simulink model "UZ_EnDat_be4_optimizing_agaib"  (R2023b)
settings: Solver=FixedStepDiscrete  StartTime=0  StopTime=0.002  RelTol=1e-3
model workspace (MAT data in the model file):
  Select = 0
libraries: hdlsllib x750, simulink x19, simulink_extras x4
(part 5 of 9)

== system UZ_EnDat_be4_optimizing_agaib/UZ_ENDAT/ManualSerialize/nibblepadding6/padding2 ==
  in : Inport
  Bit Shift2 : hdlsllib/Logic and Bit Operations/Bit Shift  mode=Shift Right Logical  N=1
  Bit Slice2 : hdlsllib/Logic and Bit Operations/Bit Slice  lidx=0  ridx=0
  Data Type Conversion2 : DataTypeConversion  OutDataTypeStr=boolean  RndMeth=Nearest  SaturateOnIntegerOverflow=off
  Switch2 : Switch  Criteria=u2 > Threshold  SaturateOnIntegerOverflow=off  InputSameDT=off
  out : Outport
  wires:
  in/1 -> Bit Shift2/1, Switch2/1, Bit Slice2/1
  Bit Shift2/1 -> Switch2/3
  Data Type Conversion2/1 -> Switch2/2
  Bit Slice2/1 -> Data Type Conversion2/1
  Switch2/1 -> out/1

== system UZ_EnDat_be4_optimizing_agaib/UZ_ENDAT/ManualSerialize/nibblepadding6/padding3 ==
  in : Inport
  Bit Shift2 : hdlsllib/Logic and Bit Operations/Bit Shift  mode=Shift Right Logical  N=1
  Bit Slice2 : hdlsllib/Logic and Bit Operations/Bit Slice  lidx=0  ridx=0
  Data Type Conversion2 : DataTypeConversion  OutDataTypeStr=boolean  RndMeth=Nearest  SaturateOnIntegerOverflow=off
  Switch2 : Switch  Criteria=u2 > Threshold  SaturateOnIntegerOverflow=off  InputSameDT=off
  out : Outport
  wires:
  in/1 -> Bit Shift2/1, Switch2/1, Bit Slice2/1
  Bit Shift2/1 -> Switch2/3
  Data Type Conversion2/1 -> Switch2/2
  Bit Slice2/1 -> Data Type Conversion2/1
  Switch2/1 -> out/1

== system UZ_EnDat_be4_optimizing_agaib/UZ_ENDAT/ManualSerialize/padder/nibblepadding1 ==
  in : Inport
  padding : Subsystem  Commented=through
  padding1 : Subsystem
  padding2 : Subsystem
  padding3 : Subsystem
  out : Outport
  wires:
  in/1 -> padding3/1(in)
  padding2/1(out) -> padding1/1(in)
  padding3/1(out) -> padding2/1(in)
  padding1/1(out) -> padding/1(in)
  padding/1(out) -> out/1

== system UZ_EnDat_be4_optimizing_agaib/UZ_ENDAT/ManualSerialize/padder/nibblepadding10 ==
  in : Inport
  padding : Subsystem  Commented=through
  padding1 : Subsystem
  padding2 : Subsystem
  padding3 : Subsystem
  out : Outport
  wires:
  in/1 -> padding3/1(in)
  padding2/1(out) -> padding1/1(in)
  padding3/1(out) -> padding2/1(in)
  padding1/1(out) -> padding/1(in)
  padding/1(out) -> out/1

== system UZ_EnDat_be4_optimizing_agaib/UZ_ENDAT/ManualSerialize/padder/nibblepadding11 ==
  in : Inport
  padding : Subsystem  Commented=through
  padding1 : Subsystem
  padding2 : Subsystem
  padding3 : Subsystem
  out : Outport
  wires:
  in/1 -> padding3/1(in)
  padding2/1(out) -> padding1/1(in)
  padding3/1(out) -> padding2/1(in)
  padding1/1(out) -> padding/1(in)
  padding/1(out) -> out/1

== system UZ_EnDat_be4_optimizing_agaib/UZ_ENDAT/ManualSerialize/padder/nibblepadding12 ==
  in : Inport
  padding : Subsystem  Commented=through
  padding1 : Subsystem
  padding2 : Subsystem
  padding3 : Subsystem
  out : Outport
  wires:
  in/1 -> padding3/1(in)
  padding2/1(out) -> padding1/1(in)
  padding3/1(out) -> padding2/1(in)
  padding1/1(out) -> padding/1(in)
  padding/1(out) -> out/1

== system UZ_EnDat_be4_optimizing_agaib/UZ_ENDAT/ManualSerialize/padder/nibblepadding13 ==
  in : Inport
  padding : Subsystem  Commented=through
  padding1 : Subsystem
  padding2 : Subsystem
  padding3 : Subsystem
  out : Outport
  wires:
  in/1 -> padding3/1(in)
  padding2/1(out) -> padding1/1(in)
  padding3/1(out) -> padding2/1(in)
  padding1/1(out) -> padding/1(in)
  padding/1(out) -> out/1

== system UZ_EnDat_be4_optimizing_agaib/UZ_ENDAT/ManualSerialize/padder/nibblepadding14 ==
  in : Inport
  padding : Subsystem  Commented=through
  padding1 : Subsystem
  padding2 : Subsystem
  padding3 : Subsystem
  out : Outport
  wires:
  in/1 -> padding3/1(in)
  padding2/1(out) -> padding1/1(in)
  padding3/1(out) -> padding2/1(in)
  padding1/1(out) -> padding/1(in)
  padding/1(out) -> out/1

== system UZ_EnDat_be4_optimizing_agaib/UZ_ENDAT/ManualSerialize/padder/nibblepadding15 ==
  in : Inport
  padding : Subsystem  Commented=through
  padding1 : Subsystem
  padding2 : Subsystem
  padding3 : Subsystem
  out : Outport
  wires:
  in/1 -> padding3/1(in)
  padding2/1(out) -> padding1/1(in)
  padding3/1(out) -> padding2/1(in)
  padding1/1(out) -> padding/1(in)
  padding/1(out) -> out/1

== system UZ_EnDat_be4_optimizing_agaib/UZ_ENDAT/ManualSerialize/padder/nibblepadding16 ==
  in : Inport
  padding : Subsystem  Commented=through
  padding1 : Subsystem
  padding2 : Subsystem
  padding3 : Subsystem
  out : Outport
  wires:
  in/1 -> padding3/1(in)
  padding2/1(out) -> padding1/1(in)
  padding3/1(out) -> padding2/1(in)
  padding1/1(out) -> padding/1(in)
  padding/1(out) -> out/1

== system UZ_EnDat_be4_optimizing_agaib/UZ_ENDAT/ManualSerialize/padder/nibblepadding17 ==
  in : Inport
  padding : Subsystem  Commented=through
  padding1 : Subsystem
  padding2 : Subsystem
  padding3 : Subsystem
  out : Outport
  wires:
  in/1 -> padding3/1(in)
  padding2/1(out) -> padding1/1(in)
  padding3/1(out) -> padding2/1(in)
  padding1/1(out) -> padding/1(in)
  padding/1(out) -> out/1

== system UZ_EnDat_be4_optimizing_agaib/UZ_ENDAT/ManualSerialize/padder/nibblepadding18 ==
  in : Inport
  padding : Subsystem  Commented=through
  padding1 : Subsystem
  padding2 : Subsystem
  padding3 : Subsystem
  out : Outport
  wires:
  in/1 -> padding3/1(in)
  padding2/1(out) -> padding1/1(in)
  padding3/1(out) -> padding2/1(in)
  padding1/1(out) -> padding/1(in)
  padding/1(out) -> out/1

== system UZ_EnDat_be4_optimizing_agaib/UZ_ENDAT/ManualSerialize/padder/nibblepadding19 ==
  in : Inport
  padding : Subsystem  Commented=through
  padding1 : Subsystem
  padding2 : Subsystem
  padding3 : Subsystem
  out : Outport
  wires:
  in/1 -> padding3/1(in)
  padding2/1(out) -> padding1/1(in)
  padding3/1(out) -> padding2/1(in)
  padding1/1(out) -> padding/1(in)
  padding/1(out) -> out/1

== system UZ_EnDat_be4_optimizing_agaib/UZ_ENDAT/ManualSerialize/padder/nibblepadding2 ==
  in : Inport
  padding : Subsystem  Commented=through
  padding1 : Subsystem
  padding2 : Subsystem
  padding3 : Subsystem
  out : Outport
  wires:
  in/1 -> padding3/1(in)
  padding2/1(out) -> padding1/1(in)
  padding3/1(out) -> padding2/1(in)
  padding1/1(out) -> padding/1(in)
  padding/1(out) -> out/1

== system UZ_EnDat_be4_optimizing_agaib/UZ_ENDAT/ManualSerialize/padder/nibblepadding20 ==
  in : Inport
  padding : Subsystem  Commented=through
  padding1 : Subsystem
  padding2 : Subsystem
  padding3 : Subsystem
  out : Outport
  wires:
  in/1 -> padding3/1(in)
  padding2/1(out) -> padding1/1(in)
  padding3/1(out) -> padding2/1(in)
  padding1/1(out) -> padding/1(in)
  padding/1(out) -> out/1

== system UZ_EnDat_be4_optimizing_agaib/UZ_ENDAT/ManualSerialize/padder/nibblepadding21 ==
  in : Inport
  padding : Subsystem  Commented=through
  padding1 : Subsystem
  padding2 : Subsystem
  padding3 : Subsystem
  out : Outport
  wires:
  in/1 -> padding3/1(in)
  padding2/1(out) -> padding1/1(in)
  padding3/1(out) -> padding2/1(in)
  padding1/1(out) -> padding/1(in)
  padding/1(out) -> out/1

== system UZ_EnDat_be4_optimizing_agaib/UZ_ENDAT/ManualSerialize/padder/nibblepadding22 ==
  in : Inport
  padding : Subsystem  Commented=through
  padding1 : Subsystem
  padding2 : Subsystem
  padding3 : Subsystem
  out : Outport
  wires:
  in/1 -> padding3/1(in)
  padding2/1(out) -> padding1/1(in)
  padding3/1(out) -> padding2/1(in)
  padding1/1(out) -> padding/1(in)
  padding/1(out) -> out/1

== system UZ_EnDat_be4_optimizing_agaib/UZ_ENDAT/ManualSerialize/padder/nibblepadding23 ==
  in : Inport
  padding : Subsystem  Commented=through
  padding1 : Subsystem
  padding2 : Subsystem
  padding3 : Subsystem
  out : Outport
  wires:
  in/1 -> padding3/1(in)
  padding2/1(out) -> padding1/1(in)
  padding3/1(out) -> padding2/1(in)
  padding1/1(out) -> padding/1(in)
  padding/1(out) -> out/1

== system UZ_EnDat_be4_optimizing_agaib/UZ_ENDAT/ManualSerialize/padder/nibblepadding24 ==
  in : Inport
  padding : Subsystem  Commented=through
  padding1 : Subsystem
  padding2 : Subsystem
  padding3 : Subsystem
  out : Outport
  wires:
  in/1 -> padding3/1(in)
  padding2/1(out) -> padding1/1(in)
  padding3/1(out) -> padding2/1(in)
  padding1/1(out) -> padding/1(in)
  padding/1(out) -> out/1

== system UZ_EnDat_be4_optimizing_agaib/UZ_ENDAT/ManualSerialize/padder/nibblepadding25 ==
  in : Inport
  padding : Subsystem  Commented=through
  padding1 : Subsystem
  padding2 : Subsystem
  padding3 : Subsystem
  out : Outport
  wires:
  in/1 -> padding3/1(in)
  padding2/1(out) -> padding1/1(in)
  padding3/1(out) -> padding2/1(in)
  padding1/1(out) -> padding/1(in)
  padding/1(out) -> out/1

== system UZ_EnDat_be4_optimizing_agaib/UZ_ENDAT/ManualSerialize/padder/nibblepadding26 ==
  in : Inport
  padding : Subsystem  Commented=through
  padding1 : Subsystem
  padding2 : Subsystem
  padding3 : Subsystem
  out : Outport
  wires:
  in/1 -> padding3/1(in)
  padding2/1(out) -> padding1/1(in)
  padding3/1(out) -> padding2/1(in)
  padding1/1(out) -> padding/1(in)
  padding/1(out) -> out/1

== system UZ_EnDat_be4_optimizing_agaib/UZ_ENDAT/ManualSerialize/padder/nibblepadding27 ==
  in : Inport
  padding : Subsystem  Commented=through
  padding1 : Subsystem
  padding2 : Subsystem
  padding3 : Subsystem
  out : Outport
  wires:
  in/1 -> padding3/1(in)
  padding2/1(out) -> padding1/1(in)
  padding3/1(out) -> padding2/1(in)
  padding1/1(out) -> padding/1(in)
  padding/1(out) -> out/1

== system UZ_EnDat_be4_optimizing_agaib/UZ_ENDAT/ManualSerialize/padder/nibblepadding28 ==
  in : Inport
  padding : Subsystem  Commented=through
  padding1 : Subsystem
  padding2 : Subsystem
  padding3 : Subsystem
  out : Outport
  wires:
  in/1 -> padding3/1(in)
  padding2/1(out) -> padding1/1(in)
  padding3/1(out) -> padding2/1(in)
  padding1/1(out) -> padding/1(in)
  padding/1(out) -> out/1

== system UZ_EnDat_be4_optimizing_agaib/UZ_ENDAT/ManualSerialize/padder/nibblepadding29 ==
  in : Inport
  padding : Subsystem  Commented=through
  padding1 : Subsystem
  padding2 : Subsystem
  padding3 : Subsystem
  out : Outport
  wires:
  in/1 -> padding3/1(in)
  padding2/1(out) -> padding1/1(in)
  padding3/1(out) -> padding2/1(in)
  padding1/1(out) -> padding/1(in)
  padding/1(out) -> out/1

== system UZ_EnDat_be4_optimizing_agaib/UZ_ENDAT/ManualSerialize/padder/nibblepadding3 ==
  in : Inport
  padding : Subsystem  Commented=through
  padding1 : Subsystem
  padding2 : Subsystem
  padding3 : Subsystem
  out : Outport
  wires:
  in/1 -> padding3/1(in)
  padding2/1(out) -> padding1/1(in)
  padding3/1(out) -> padding2/1(in)
  padding1/1(out) -> padding/1(in)
  padding/1(out) -> out/1

== system UZ_EnDat_be4_optimizing_agaib/UZ_ENDAT/ManualSerialize/padder/nibblepadding30 ==
  in : Inport
  padding : Subsystem  Commented=through
  padding1 : Subsystem
  padding2 : Subsystem
  padding3 : Subsystem
  out : Outport
  wires:
  in/1 -> padding3/1(in)
  padding2/1(out) -> padding1/1(in)
  padding3/1(out) -> padding2/1(in)
  padding1/1(out) -> padding/1(in)
  padding/1(out) -> out/1

== system UZ_EnDat_be4_optimizing_agaib/UZ_ENDAT/ManualSerialize/padder/nibblepadding4 ==
  in : Inport
  padding : Subsystem  Commented=through
  padding1 : Subsystem
  padding2 : Subsystem
  padding3 : Subsystem
  out : Outport
  wires:
  in/1 -> padding3/1(in)
  padding2/1(out) -> padding1/1(in)
  padding3/1(out) -> padding2/1(in)
  padding1/1(out) -> padding/1(in)
  padding/1(out) -> out/1

== system UZ_EnDat_be4_optimizing_agaib/UZ_ENDAT/ManualSerialize/padder/nibblepadding5 ==
  in : Inport
  padding : Subsystem  Commented=through
  padding1 : Subsystem
  padding2 : Subsystem
  padding3 : Subsystem
  out : Outport
  wires:
  in/1 -> padding3/1(in)
  padding2/1(out) -> padding1/1(in)
  padding3/1(out) -> padding2/1(in)
  padding1/1(out) -> padding/1(in)
  padding/1(out) -> out/1

== system UZ_EnDat_be4_optimizing_agaib/UZ_ENDAT/ManualSerialize/padder/nibblepadding6 ==
  in : Inport
  padding : Subsystem  Commented=through
  padding1 : Subsystem
  padding2 : Subsystem
  padding3 : Subsystem
  out : Outport
  wires:
  in/1 -> padding3/1(in)
  padding2/1(out) -> padding1/1(in)
  padding3/1(out) -> padding2/1(in)
  padding1/1(out) -> padding/1(in)
  padding/1(out) -> out/1

== system UZ_EnDat_be4_optimizing_agaib/UZ_ENDAT/ManualSerialize/padder/nibblepadding7 ==
  in : Inport
  padding : Subsystem  Commented=through
  padding1 : Subsystem
  padding2 : Subsystem
  padding3 : Subsystem
  out : Outport
  wires:
  in/1 -> padding3/1(in)
  padding2/1(out) -> padding1/1(in)
  padding3/1(out) -> padding2/1(in)
  padding1/1(out) -> padding/1(in)
  padding/1(out) -> out/1

== system UZ_EnDat_be4_optimizing_agaib/UZ_ENDAT/ManualSerialize/padder/nibblepadding8 ==
  in : Inport
  padding : Subsystem  Commented=through
  padding1 : Subsystem
  padding2 : Subsystem
  padding3 : Subsystem
  out : Outport
  wires:
  in/1 -> padding3/1(in)
  padding2/1(out) -> padding1/1(in)
  padding3/1(out) -> padding2/1(in)
  padding1/1(out) -> padding/1(in)
  padding/1(out) -> out/1

== system UZ_EnDat_be4_optimizing_agaib/UZ_ENDAT/ManualSerialize/padder/nibblepadding9 ==
  in : Inport
  padding : Subsystem  Commented=through
  padding1 : Subsystem
  padding2 : Subsystem
  padding3 : Subsystem
  out : Outport
  wires:
  in/1 -> padding3/1(in)
  padding2/1(out) -> padding1/1(in)
  padding3/1(out) -> padding2/1(in)
  padding1/1(out) -> padding/1(in)
  padding/1(out) -> out/1

== system UZ_EnDat_be4_optimizing_agaib/UZ_ENDAT/ManualSerialize1/Storage1/prolonger ==
  in : Inport
  Delay4 : Delay  DelayLength=1
  Logical Operator5 : Logic  Operator=OR  AllPortsSameDT=off  OutDataTypeStr=boolean
  out : Outport
  wires:
  Logical Operator5/1 -> out/1
  in/1 -> Delay4/1, Logical Operator5/1
  Delay4/1 -> Logical Operator5/2

== system UZ_EnDat_be4_optimizing_agaib/UZ_ENDAT/ManualSerialize1/Storage2/prolonger ==
  in : Inport
  Delay4 : Delay  DelayLength=1
  Logical Operator5 : Logic  Operator=OR  Inputs=3  AllPortsSameDT=off  OutDataTypeStr=boolean
  out : Outport
  wires:
  Logical Operator5/1 -> out/1
  in/1 -> Logical Operator5/3, Delay4/1, Logical Operator5/1
  Delay4/1 -> Logical Operator5/2

== system UZ_EnDat_be4_optimizing_agaib/UZ_ENDAT/ManualSerialize1/nibblepadding6/padding ==
  in : Inport
  Bit Shift2 : hdlsllib/Logic and Bit Operations/Bit Shift  mode=Shift Right Logical  N=1
  Bit Slice2 : hdlsllib/Logic and Bit Operations/Bit Slice  lidx=0  ridx=0
  Data Type Conversion2 : DataTypeConversion  OutDataTypeStr=boolean  RndMeth=Nearest  SaturateOnIntegerOverflow=off
  Switch2 : Switch  Criteria=u2 > Threshold  SaturateOnIntegerOverflow=off  InputSameDT=off
  out : Outport
  wires:
  in/1 -> Bit Shift2/1, Switch2/1, Bit Slice2/1
  Bit Shift2/1 -> Switch2/3
  Data Type Conversion2/1 -> Switch2/2
  Bit Slice2/1 -> Data Type Conversion2/1
  Switch2/1 -> out/1

== system UZ_EnDat_be4_optimizing_agaib/UZ_ENDAT/ManualSerialize1/nibblepadding6/padding1 ==
  in : Inport
  Bit Shift2 : hdlsllib/Logic and Bit Operations/Bit Shift  mode=Shift Right Logical  N=1
  Bit Slice2 : hdlsllib/Logic and Bit Operations/Bit Slice  lidx=0  ridx=0
  Data Type Conversion2 : DataTypeConversion  OutDataTypeStr=boolean  RndMeth=Nearest  SaturateOnIntegerOverflow=off
  Switch2 : Switch  Criteria=u2 > Threshold  SaturateOnIntegerOverflow=off  InputSameDT=off
  out : Outport
  wires:
  in/1 -> Bit Shift2/1, Switch2/1, Bit Slice2/1
  Bit Shift2/1 -> Switch2/3
  Data Type Conversion2/1 -> Switch2/2
  Bit Slice2/1 -> Data Type Conversion2/1
  Switch2/1 -> out/1

== system UZ_EnDat_be4_optimizing_agaib/UZ_ENDAT/ManualSerialize1/nibblepadding6/padding2 ==
  in : Inport
  Bit Shift2 : hdlsllib/Logic and Bit Operations/Bit Shift  mode=Shift Right Logical  N=1
  Bit Slice2 : hdlsllib/Logic and Bit Operations/Bit Slice  lidx=0  ridx=0
  Data Type Conversion2 : DataTypeConversion  OutDataTypeStr=boolean  RndMeth=Nearest  SaturateOnIntegerOverflow=off
  Switch2 : Switch  Criteria=u2 > Threshold  SaturateOnIntegerOverflow=off  InputSameDT=off
  out : Outport
  wires:
  in/1 -> Bit Shift2/1, Switch2/1, Bit Slice2/1
  Bit Shift2/1 -> Switch2/3
  Data Type Conversion2/1 -> Switch2/2
  Bit Slice2/1 -> Data Type Conversion2/1
  Switch2/1 -> out/1

== system UZ_EnDat_be4_optimizing_agaib/UZ_ENDAT/ManualSerialize1/nibblepadding6/padding3 ==
  in : Inport
  Bit Shift2 : hdlsllib/Logic and Bit Operations/Bit Shift  mode=Shift Right Logical  N=1
  Bit Slice2 : hdlsllib/Logic and Bit Operations/Bit Slice  lidx=0  ridx=0
  Data Type Conversion2 : DataTypeConversion  OutDataTypeStr=boolean  RndMeth=Nearest  SaturateOnIntegerOverflow=off
  Switch2 : Switch  Criteria=u2 > Threshold  SaturateOnIntegerOverflow=off  InputSameDT=off
  out : Outport
  wires:
  in/1 -> Bit Shift2/1, Switch2/1, Bit Slice2/1
  Bit Shift2/1 -> Switch2/3
  Data Type Conversion2/1 -> Switch2/2
  Bit Slice2/1 -> Data Type Conversion2/1
  Switch2/1 -> out/1

== system UZ_EnDat_be4_optimizing_agaib/UZ_ENDAT/ManualSerialize1/padder/nibblepadding1 ==
  in : Inport
  padding : Subsystem  Commented=through
  padding1 : Subsystem
  padding2 : Subsystem
  padding3 : Subsystem
  out : Outport
  wires:
  in/1 -> padding3/1(in)
  padding2/1(out) -> padding1/1(in)
  padding3/1(out) -> padding2/1(in)
  padding1/1(out) -> padding/1(in)
  padding/1(out) -> out/1

== system UZ_EnDat_be4_optimizing_agaib/UZ_ENDAT/ManualSerialize1/padder/nibblepadding10 ==
  in : Inport
  padding : Subsystem  Commented=through
  padding1 : Subsystem
  padding2 : Subsystem
  padding3 : Subsystem
  out : Outport
  wires:
  in/1 -> padding3/1(in)
  padding2/1(out) -> padding1/1(in)
  padding3/1(out) -> padding2/1(in)
  padding1/1(out) -> padding/1(in)
  padding/1(out) -> out/1

== system UZ_EnDat_be4_optimizing_agaib/UZ_ENDAT/ManualSerialize1/padder/nibblepadding11 ==
  in : Inport
  padding : Subsystem  Commented=through
  padding1 : Subsystem
  padding2 : Subsystem
  padding3 : Subsystem
  out : Outport
  wires:
  in/1 -> padding3/1(in)
  padding2/1(out) -> padding1/1(in)
  padding3/1(out) -> padding2/1(in)
  padding1/1(out) -> padding/1(in)
  padding/1(out) -> out/1

== system UZ_EnDat_be4_optimizing_agaib/UZ_ENDAT/ManualSerialize1/padder/nibblepadding12 ==
  in : Inport
  padding : Subsystem  Commented=through
  padding1 : Subsystem
  padding2 : Subsystem
  padding3 : Subsystem
  out : Outport
  wires:
  in/1 -> padding3/1(in)
  padding2/1(out) -> padding1/1(in)
  padding3/1(out) -> padding2/1(in)
  padding1/1(out) -> padding/1(in)
  padding/1(out) -> out/1

== system UZ_EnDat_be4_optimizing_agaib/UZ_ENDAT/ManualSerialize1/padder/nibblepadding13 ==
  in : Inport
  padding : Subsystem  Commented=through
  padding1 : Subsystem
  padding2 : Subsystem
  padding3 : Subsystem
  out : Outport
  wires:
  in/1 -> padding3/1(in)
  padding2/1(out) -> padding1/1(in)
  padding3/1(out) -> padding2/1(in)
  padding1/1(out) -> padding/1(in)
  padding/1(out) -> out/1

== system UZ_EnDat_be4_optimizing_agaib/UZ_ENDAT/ManualSerialize1/padder/nibblepadding14 ==
  in : Inport
  padding : Subsystem  Commented=through
  padding1 : Subsystem
  padding2 : Subsystem
  padding3 : Subsystem
  out : Outport
  wires:
  in/1 -> padding3/1(in)
  padding2/1(out) -> padding1/1(in)
  padding3/1(out) -> padding2/1(in)
  padding1/1(out) -> padding/1(in)
  padding/1(out) -> out/1

== system UZ_EnDat_be4_optimizing_agaib/UZ_ENDAT/ManualSerialize1/padder/nibblepadding15 ==
  in : Inport
  padding : Subsystem  Commented=through
  padding1 : Subsystem
  padding2 : Subsystem
  padding3 : Subsystem
  out : Outport
  wires:
  in/1 -> padding3/1(in)
  padding2/1(out) -> padding1/1(in)
  padding3/1(out) -> padding2/1(in)
  padding1/1(out) -> padding/1(in)
  padding/1(out) -> out/1

== system UZ_EnDat_be4_optimizing_agaib/UZ_ENDAT/ManualSerialize1/padder/nibblepadding16 ==
  in : Inport
  padding : Subsystem  Commented=through
  padding1 : Subsystem
  padding2 : Subsystem
  padding3 : Subsystem
  out : Outport
  wires:
  in/1 -> padding3/1(in)
  padding2/1(out) -> padding1/1(in)
  padding3/1(out) -> padding2/1(in)
  padding1/1(out) -> padding/1(in)
  padding/1(out) -> out/1

== system UZ_EnDat_be4_optimizing_agaib/UZ_ENDAT/ManualSerialize1/padder/nibblepadding17 ==
  in : Inport
  padding : Subsystem  Commented=through
  padding1 : Subsystem
  padding2 : Subsystem
  padding3 : Subsystem
  out : Outport
  wires:
  in/1 -> padding3/1(in)
  padding2/1(out) -> padding1/1(in)
  padding3/1(out) -> padding2/1(in)
  padding1/1(out) -> padding/1(in)
  padding/1(out) -> out/1

== system UZ_EnDat_be4_optimizing_agaib/UZ_ENDAT/ManualSerialize1/padder/nibblepadding18 ==
  in : Inport
  padding : Subsystem  Commented=through
  padding1 : Subsystem
  padding2 : Subsystem
  padding3 : Subsystem
  out : Outport
  wires:
  in/1 -> padding3/1(in)
  padding2/1(out) -> padding1/1(in)
  padding3/1(out) -> padding2/1(in)
  padding1/1(out) -> padding/1(in)
  padding/1(out) -> out/1

== system UZ_EnDat_be4_optimizing_agaib/UZ_ENDAT/ManualSerialize1/padder/nibblepadding19 ==
  in : Inport
  padding : Subsystem  Commented=through
  padding1 : Subsystem
  padding2 : Subsystem
  padding3 : Subsystem
  out : Outport
  wires:
  in/1 -> padding3/1(in)
  padding2/1(out) -> padding1/1(in)
  padding3/1(out) -> padding2/1(in)
  padding1/1(out) -> padding/1(in)
  padding/1(out) -> out/1

== system UZ_EnDat_be4_optimizing_agaib/UZ_ENDAT/ManualSerialize1/padder/nibblepadding2 ==
  in : Inport
  padding : Subsystem  Commented=through
  padding1 : Subsystem
  padding2 : Subsystem
  padding3 : Subsystem
  out : Outport
  wires:
  in/1 -> padding3/1(in)
  padding2/1(out) -> padding1/1(in)
  padding3/1(out) -> padding2/1(in)
  padding1/1(out) -> padding/1(in)
  padding/1(out) -> out/1

== system UZ_EnDat_be4_optimizing_agaib/UZ_ENDAT/ManualSerialize1/padder/nibblepadding20 ==
  in : Inport
  padding : Subsystem  Commented=through
  padding1 : Subsystem
  padding2 : Subsystem
  padding3 : Subsystem
  out : Outport
  wires:
  in/1 -> padding3/1(in)
  padding2/1(out) -> padding1/1(in)
  padding3/1(out) -> padding2/1(in)
  padding1/1(out) -> padding/1(in)
  padding/1(out) -> out/1

== system UZ_EnDat_be4_optimizing_agaib/UZ_ENDAT/ManualSerialize1/padder/nibblepadding21 ==
  in : Inport
  padding : Subsystem  Commented=through
  padding1 : Subsystem
  padding2 : Subsystem
  padding3 : Subsystem
  out : Outport
  wires:
  in/1 -> padding3/1(in)
  padding2/1(out) -> padding1/1(in)
  padding3/1(out) -> padding2/1(in)
  padding1/1(out) -> padding/1(in)
  padding/1(out) -> out/1

== system UZ_EnDat_be4_optimizing_agaib/UZ_ENDAT/ManualSerialize1/padder/nibblepadding22 ==
  in : Inport
  padding : Subsystem  Commented=through
  padding1 : Subsystem
  padding2 : Subsystem
  padding3 : Subsystem
  out : Outport
  wires:
  in/1 -> padding3/1(in)
  padding2/1(out) -> padding1/1(in)
  padding3/1(out) -> padding2/1(in)
  padding1/1(out) -> padding/1(in)
  padding/1(out) -> out/1

== system UZ_EnDat_be4_optimizing_agaib/UZ_ENDAT/ManualSerialize1/padder/nibblepadding23 ==
  in : Inport
  padding : Subsystem  Commented=through
  padding1 : Subsystem
  padding2 : Subsystem
  padding3 : Subsystem
  out : Outport
  wires:
  in/1 -> padding3/1(in)
  padding2/1(out) -> padding1/1(in)
  padding3/1(out) -> padding2/1(in)
  padding1/1(out) -> padding/1(in)
  padding/1(out) -> out/1

== system UZ_EnDat_be4_optimizing_agaib/UZ_ENDAT/ManualSerialize1/padder/nibblepadding24 ==
  in : Inport
  padding : Subsystem  Commented=through
  padding1 : Subsystem
  padding2 : Subsystem
  padding3 : Subsystem
  out : Outport
  wires:
  in/1 -> padding3/1(in)
  padding2/1(out) -> padding1/1(in)
  padding3/1(out) -> padding2/1(in)
  padding1/1(out) -> padding/1(in)
  padding/1(out) -> out/1

== system UZ_EnDat_be4_optimizing_agaib/UZ_ENDAT/ManualSerialize1/padder/nibblepadding25 ==
  in : Inport
  padding : Subsystem  Commented=through
  padding1 : Subsystem
  padding2 : Subsystem
  padding3 : Subsystem
  out : Outport
  wires:
  in/1 -> padding3/1(in)
  padding2/1(out) -> padding1/1(in)
  padding3/1(out) -> padding2/1(in)
  padding1/1(out) -> padding/1(in)
  padding/1(out) -> out/1

== system UZ_EnDat_be4_optimizing_agaib/UZ_ENDAT/ManualSerialize1/padder/nibblepadding26 ==
  in : Inport
  padding : Subsystem  Commented=through
  padding1 : Subsystem
  padding2 : Subsystem
  padding3 : Subsystem
  out : Outport
  wires:
  in/1 -> padding3/1(in)
  padding2/1(out) -> padding1/1(in)
  padding3/1(out) -> padding2/1(in)
  padding1/1(out) -> padding/1(in)
  padding/1(out) -> out/1

== system UZ_EnDat_be4_optimizing_agaib/UZ_ENDAT/ManualSerialize1/padder/nibblepadding27 ==
  in : Inport
  padding : Subsystem  Commented=through
  padding1 : Subsystem
  padding2 : Subsystem
  padding3 : Subsystem
  out : Outport
  wires:
  in/1 -> padding3/1(in)
  padding2/1(out) -> padding1/1(in)
  padding3/1(out) -> padding2/1(in)
  padding1/1(out) -> padding/1(in)
  padding/1(out) -> out/1

== system UZ_EnDat_be4_optimizing_agaib/UZ_ENDAT/ManualSerialize1/padder/nibblepadding28 ==
  in : Inport
  padding : Subsystem  Commented=through
  padding1 : Subsystem
  padding2 : Subsystem
  padding3 : Subsystem
  out : Outport
  wires:
  in/1 -> padding3/1(in)
  padding2/1(out) -> padding1/1(in)
  padding3/1(out) -> padding2/1(in)
  padding1/1(out) -> padding/1(in)
  padding/1(out) -> out/1

== system UZ_EnDat_be4_optimizing_agaib/UZ_ENDAT/ManualSerialize1/padder/nibblepadding29 ==
  in : Inport
  padding : Subsystem  Commented=through
  padding1 : Subsystem
  padding2 : Subsystem
  padding3 : Subsystem
  out : Outport
  wires:
  in/1 -> padding3/1(in)
  padding2/1(out) -> padding1/1(in)
  padding3/1(out) -> padding2/1(in)
  padding1/1(out) -> padding/1(in)
  padding/1(out) -> out/1

== system UZ_EnDat_be4_optimizing_agaib/UZ_ENDAT/ManualSerialize1/padder/nibblepadding3 ==
  in : Inport
  padding : Subsystem  Commented=through
  padding1 : Subsystem
  padding2 : Subsystem
  padding3 : Subsystem
  out : Outport
  wires:
  in/1 -> padding3/1(in)
  padding2/1(out) -> padding1/1(in)
  padding3/1(out) -> padding2/1(in)
  padding1/1(out) -> padding/1(in)
  padding/1(out) -> out/1

== system UZ_EnDat_be4_optimizing_agaib/UZ_ENDAT/ManualSerialize1/padder/nibblepadding4 ==
  in : Inport
  padding : Subsystem  Commented=through
  padding1 : Subsystem
  padding2 : Subsystem
  padding3 : Subsystem
  out : Outport
  wires:
  in/1 -> padding3/1(in)
  padding2/1(out) -> padding1/1(in)
  padding3/1(out) -> padding2/1(in)
  padding1/1(out) -> padding/1(in)
  padding/1(out) -> out/1

== system UZ_EnDat_be4_optimizing_agaib/UZ_ENDAT/ManualSerialize1/padder/nibblepadding5 ==
  in : Inport
  padding : Subsystem  Commented=through
  padding1 : Subsystem
  padding2 : Subsystem
  padding3 : Subsystem
  out : Outport
  wires:
  in/1 -> padding3/1(in)
  padding2/1(out) -> padding1/1(in)
  padding3/1(out) -> padding2/1(in)
  padding1/1(out) -> padding/1(in)
  padding/1(out) -> out/1

== system UZ_EnDat_be4_optimizing_agaib/UZ_ENDAT/ManualSerialize1/padder/nibblepadding6 ==
  in : Inport
  padding : Subsystem  Commented=through
  padding1 : Subsystem
  padding2 : Subsystem
  padding3 : Subsystem
  out : Outport
  wires:
  in/1 -> padding3/1(in)
  padding2/1(out) -> padding1/1(in)
  padding3/1(out) -> padding2/1(in)
  padding1/1(out) -> padding/1(in)
  padding/1(out) -> out/1

== system UZ_EnDat_be4_optimizing_agaib/UZ_ENDAT/ManualSerialize1/padder/nibblepadding7 ==
  in : Inport
  padding : Subsystem  Commented=through
  padding1 : Subsystem
  padding2 : Subsystem
  padding3 : Subsystem
  out : Outport
  wires:
  in/1 -> padding3/1(in)
  padding2/1(out) -> padding1/1(in)
  padding3/1(out) -> padding2/1(in)
  padding1/1(out) -> padding/1(in)
  padding/1(out) -> out/1

== system UZ_EnDat_be4_optimizing_agaib/UZ_ENDAT/ManualSerialize1/padder/nibblepadding8 ==
  in : Inport
  padding : Subsystem  Commented=through
  padding1 : Subsystem
  padding2 : Subsystem
  padding3 : Subsystem
  out : Outport
  wires:
  in/1 -> padding3/1(in)
  padding2/1(out) -> padding1/1(in)
  padding3/1(out) -> padding2/1(in)
  padding1/1(out) -> padding/1(in)
  padding/1(out) -> out/1

== system UZ_EnDat_be4_optimizing_agaib/UZ_ENDAT/ManualSerialize1/padder/nibblepadding9 ==
  in : Inport
  padding : Subsystem  Commented=through
  padding1 : Subsystem
  padding2 : Subsystem
  padding3 : Subsystem
  out : Outport
  wires:
  in/1 -> padding3/1(in)
  padding2/1(out) -> padding1/1(in)
  padding3/1(out) -> padding2/1(in)
  padding1/1(out) -> padding/1(in)
  padding/1(out) -> out/1

== system UZ_EnDat_be4_optimizing_agaib/UZ_ENDAT/RESPONSESLICER3X/19BITSLICER/responseslicer ==
  DATA : Inport  OutDataTypeStr=uint64
  Bit Slice1 : hdlsllib/Logic and Bit Operations/Bit Slice  lidx=2  ridx=2
  Bit Slice3 : hdlsllib/Logic and Bit Operations/Bit Slice  lidx=25  ridx=21
  Bit Slice4 : hdlsllib/Logic and Bit Operations/Bit Slice  lidx=20  ridx=2
  Data Type Conversion1 : DataTypeConversion  OutDataTypeStr=boolean  SaturateOnIntegerOverflow=off  RndMeth=Floor
  Data Type Conversion3 : DataTypeConversion  OutDataTypeStr=uint8  SaturateOnIntegerOverflow=off  RndMeth=Floor
  Data Type Conversion4 : DataTypeConversion  OutDataTypeStr=uint32  SaturateOnIntegerOverflow=off  RndMeth=Floor
  Terminator : Terminator
  CRC : Outport  OutDataTypeStr=uint8
  payload : Outport  Port=2  OutDataTypeStr=uint32
  error : Outport  Port=3  OutDataTypeStr=boolean
  wires:
  DATA/1 -> Terminator/1, Bit Slice1/1, Bit Slice4/1, Bit Slice3/1
  Bit Slice3/1 -> Data Type Conversion3/1
  Bit Slice4/1 -> Data Type Conversion4/1
  Data Type Conversion3/1 -> CRC/1
  Data Type Conversion4/1 -> payload/1
  Bit Slice1/1 -> Data Type Conversion1/1
  Data Type Conversion1/1 -> error/1

== system UZ_EnDat_be4_optimizing_agaib/UZ_ENDAT/RESPONSESLICER3X/19BITSLICER/responseslicer1 ==
  DATA : Inport  OutDataTypeStr=uint64
  Bit Slice1 : hdlsllib/Logic and Bit Operations/Bit Slice  lidx=2  ridx=2
  Bit Slice3 : hdlsllib/Logic and Bit Operations/Bit Slice  lidx=25  ridx=21
  Bit Slice4 : hdlsllib/Logic and Bit Operations/Bit Slice  lidx=20  ridx=2
  Data Type Conversion1 : DataTypeConversion  OutDataTypeStr=boolean  SaturateOnIntegerOverflow=off  RndMeth=Floor
  Data Type Conversion3 : DataTypeConversion  OutDataTypeStr=uint8  SaturateOnIntegerOverflow=off  RndMeth=Floor
  Data Type Conversion4 : DataTypeConversion  OutDataTypeStr=uint32  SaturateOnIntegerOverflow=off  RndMeth=Floor
  Terminator : Terminator
  CRC : Outport  OutDataTypeStr=uint8
  payload : Outport  Port=2  OutDataTypeStr=uint32
  error : Outport  Port=3  OutDataTypeStr=boolean
  wires:
  DATA/1 -> Terminator/1, Bit Slice1/1, Bit Slice4/1, Bit Slice3/1
  Bit Slice3/1 -> Data Type Conversion3/1
  Bit Slice4/1 -> Data Type Conversion4/1
  Data Type Conversion3/1 -> CRC/1
  Data Type Conversion4/1 -> payload/1
  Bit Slice1/1 -> Data Type Conversion1/1
  Data Type Conversion1/1 -> error/1

== system UZ_EnDat_be4_optimizing_agaib/UZ_ENDAT/RESPONSESLICER3X/19BITSLICER/responseslicer2 ==
  DATA : Inport  OutDataTypeStr=uint64
  Bit Slice1 : hdlsllib/Logic and Bit Operations/Bit Slice  lidx=2  ridx=2
  Bit Slice3 : hdlsllib/Logic and Bit Operations/Bit Slice  lidx=25  ridx=21
  Bit Slice4 : hdlsllib/Logic and Bit Operations/Bit Slice  lidx=20  ridx=2
  Data Type Conversion1 : DataTypeConversion  OutDataTypeStr=boolean  SaturateOnIntegerOverflow=off  RndMeth=Floor
  Data Type Conversion3 : DataTypeConversion  OutDataTypeStr=uint8  SaturateOnIntegerOverflow=off  RndMeth=Floor
  Data Type Conversion4 : DataTypeConversion  OutDataTypeStr=uint32  SaturateOnIntegerOverflow=off  RndMeth=Floor
  Terminator : Terminator
  CRC : Outport  OutDataTypeStr=uint8
  payload : Outport  Port=2  OutDataTypeStr=uint32
  error : Outport  Port=3  OutDataTypeStr=boolean
  wires:
  DATA/1 -> Terminator/1, Bit Slice1/1, Bit Slice4/1, Bit Slice3/1
  Bit Slice3/1 -> Data Type Conversion3/1
  Bit Slice4/1 -> Data Type Conversion4/1
  Data Type Conversion3/1 -> CRC/1
  Data Type Conversion4/1 -> payload/1
  Bit Slice1/1 -> Data Type Conversion1/1
  Data Type Conversion1/1 -> error/1

== system UZ_EnDat_be4_optimizing_agaib/UZ_ENDAT/RESPONSESLICER3X/21BITSLICER/responseslicer ==
  DATA : Inport  OutDataTypeStr=uint64
  Bit Slice1 : hdlsllib/Logic and Bit Operations/Bit Slice  lidx=2  ridx=2
  Bit Slice3 : hdlsllib/Logic and Bit Operations/Bit Slice  lidx=27  ridx=23
  Bit Slice4 : hdlsllib/Logic and Bit Operations/Bit Slice  lidx=22  ridx=2
  Data Type Conversion1 : DataTypeConversion  OutDataTypeStr=boolean  SaturateOnIntegerOverflow=off  RndMeth=Floor
  Data Type Conversion3 : DataTypeConversion  OutDataTypeStr=uint8  SaturateOnIntegerOverflow=off  RndMeth=Floor
  Data Type Conversion4 : DataTypeConversion  OutDataTypeStr=uint32  SaturateOnIntegerOverflow=off  RndMeth=Floor
  Terminator : Terminator
  CRC : Outport  OutDataTypeStr=uint8
  payload : Outport  Port=2  OutDataTypeStr=uint32
  error : Outport  Port=3  OutDataTypeStr=boolean
  wires:
  DATA/1 -> Terminator/1, Bit Slice1/1, Bit Slice4/1, Bit Slice3/1
  Bit Slice3/1 -> Data Type Conversion3/1
  Bit Slice4/1 -> Data Type Conversion4/1
  Data Type Conversion3/1 -> CRC/1
  Data Type Conversion4/1 -> payload/1
  Bit Slice1/1 -> Data Type Conversion1/1
  Data Type Conversion1/1 -> error/1

== system UZ_EnDat_be4_optimizing_agaib/UZ_ENDAT/RESPONSESLICER3X/21BITSLICER/responseslicer3 ==
  DATA : Inport  OutDataTypeStr=uint64
  Bit Slice1 : hdlsllib/Logic and Bit Operations/Bit Slice  lidx=2  ridx=2
  Bit Slice3 : hdlsllib/Logic and Bit Operations/Bit Slice  lidx=27  ridx=23
  Bit Slice4 : hdlsllib/Logic and Bit Operations/Bit Slice  lidx=22  ridx=2
  Data Type Conversion1 : DataTypeConversion  OutDataTypeStr=boolean  SaturateOnIntegerOverflow=off  RndMeth=Floor
  Data Type Conversion3 : DataTypeConversion  OutDataTypeStr=uint8  SaturateOnIntegerOverflow=off  RndMeth=Floor
  Data Type Conversion4 : DataTypeConversion  OutDataTypeStr=uint32  SaturateOnIntegerOverflow=off  RndMeth=Floor
  Terminator : Terminator
  CRC : Outport  OutDataTypeStr=uint8
  payload : Outport  Port=2  OutDataTypeStr=uint32
  error : Outport  Port=3  OutDataTypeStr=boolean
  wires:
  DATA/1 -> Terminator/1, Bit Slice1/1, Bit Slice4/1, Bit Slice3/1
  Bit Slice3/1 -> Data Type Conversion3/1
  Bit Slice4/1 -> Data Type Conversion4/1
  Data Type Conversion3/1 -> CRC/1
  Data Type Conversion4/1 -> payload/1
  Bit Slice1/1 -> Data Type Conversion1/1
  Data Type Conversion1/1 -> error/1

== system UZ_EnDat_be4_optimizing_agaib/UZ_ENDAT/RESPONSESLICER3X/21BITSLICER/responseslicer4 ==
  DATA : Inport  OutDataTypeStr=uint64
  Bit Slice1 : hdlsllib/Logic and Bit Operations/Bit Slice  lidx=2  ridx=2
  Bit Slice3 : hdlsllib/Logic and Bit Operations/Bit Slice  lidx=27  ridx=23
  Bit Slice4 : hdlsllib/Logic and Bit Operations/Bit Slice  lidx=22  ridx=2
  Data Type Conversion1 : DataTypeConversion  OutDataTypeStr=boolean  SaturateOnIntegerOverflow=off  RndMeth=Floor
  Data Type Conversion3 : DataTypeConversion  OutDataTypeStr=uint8  SaturateOnIntegerOverflow=off  RndMeth=Floor
  Data Type Conversion4 : DataTypeConversion  OutDataTypeStr=uint32  SaturateOnIntegerOverflow=off  RndMeth=Floor
  Terminator : Terminator
  CRC : Outport  OutDataTypeStr=uint8
  payload : Outport  Port=2  OutDataTypeStr=uint32
  error : Outport  Port=3  OutDataTypeStr=boolean
  wires:
  DATA/1 -> Terminator/1, Bit Slice1/1, Bit Slice4/1, Bit Slice3/1
  Bit Slice3/1 -> Data Type Conversion3/1
  Bit Slice4/1 -> Data Type Conversion4/1
  Data Type Conversion3/1 -> CRC/1
  Data Type Conversion4/1 -> payload/1
  Bit Slice1/1 -> Data Type Conversion1/1
  Data Type Conversion1/1 -> error/1

== system UZ_EnDat_be4_optimizing_agaib/UZ_ENDAT/RESPONSESLICER3X/23BITSLICER/responseslicer ==
  DATA : Inport  OutDataTypeStr=uint64
  Bit Slice1 : hdlsllib/Logic and Bit Operations/Bit Slice  lidx=2  ridx=2
  Bit Slice3 : hdlsllib/Logic and Bit Operations/Bit Slice  lidx=29  ridx=25
  Bit Slice4 : hdlsllib/Logic and Bit Operations/Bit Slice  lidx=24  ridx=2
  Data Type Conversion1 : DataTypeConversion  OutDataTypeStr=boolean  SaturateOnIntegerOverflow=off  RndMeth=Floor
  Data Type Conversion3 : DataTypeConversion  OutDataTypeStr=uint8  SaturateOnIntegerOverflow=off  RndMeth=Floor
  Data Type Conversion4 : DataTypeConversion  OutDataTypeStr=uint32  SaturateOnIntegerOverflow=off  RndMeth=Floor
  Terminator : Terminator
  CRC : Outport  OutDataTypeStr=uint8
  payload : Outport  Port=2  OutDataTypeStr=uint32
  error : Outport  Port=3  OutDataTypeStr=boolean
  wires:
  DATA/1 -> Terminator/1, Bit Slice1/1, Bit Slice4/1, Bit Slice3/1
  Bit Slice3/1 -> Data Type Conversion3/1
  Bit Slice4/1 -> Data Type Conversion4/1
  Data Type Conversion3/1 -> CRC/1
  Data Type Conversion4/1 -> payload/1
  Bit Slice1/1 -> Data Type Conversion1/1
  Data Type Conversion1/1 -> error/1

== system UZ_EnDat_be4_optimizing_agaib/UZ_ENDAT/RESPONSESLICER3X/23BITSLICER/responseslicer1 ==
  DATA : Inport  OutDataTypeStr=uint64
  Bit Slice1 : hdlsllib/Logic and Bit Operations/Bit Slice  lidx=2  ridx=2
  Bit Slice3 : hdlsllib/Logic and Bit Operations/Bit Slice  lidx=29  ridx=25
  Bit Slice4 : hdlsllib/Logic and Bit Operations/Bit Slice  lidx=24  ridx=2
  Data Type Conversion1 : DataTypeConversion  OutDataTypeStr=boolean  SaturateOnIntegerOverflow=off  RndMeth=Floor
  Data Type Conversion3 : DataTypeConversion  OutDataTypeStr=uint8  SaturateOnIntegerOverflow=off  RndMeth=Floor
  Data Type Conversion4 : DataTypeConversion  OutDataTypeStr=uint32  SaturateOnIntegerOverflow=off  RndMeth=Floor
  Terminator : Terminator
  CRC : Outport  OutDataTypeStr=uint8
  payload : Outport  Port=2  OutDataTypeStr=uint32
  error : Outport  Port=3  OutDataTypeStr=boolean
  wires:
  DATA/1 -> Terminator/1, Bit Slice1/1, Bit Slice4/1, Bit Slice3/1
  Bit Slice3/1 -> Data Type Conversion3/1
  Bit Slice4/1 -> Data Type Conversion4/1
  Data Type Conversion3/1 -> CRC/1
  Data Type Conversion4/1 -> payload/1
  Bit Slice1/1 -> Data Type Conversion1/1
  Data Type Conversion1/1 -> error/1

== system UZ_EnDat_be4_optimizing_agaib/UZ_ENDAT/RESPONSESLICER3X/23BITSLICER/responseslicer2 ==
  DATA : Inport  OutDataTypeStr=uint64
  Bit Slice1 : hdlsllib/Logic and Bit Operations/Bit Slice  lidx=2  ridx=2
  Bit Slice3 : hdlsllib/Logic and Bit Operations/Bit Slice  lidx=29  ridx=25
  Bit Slice4 : hdlsllib/Logic and Bit Operations/Bit Slice  lidx=24  ridx=2
  Data Type Conversion1 : DataTypeConversion  OutDataTypeStr=boolean  SaturateOnIntegerOverflow=off  RndMeth=Floor
  Data Type Conversion3 : DataTypeConversion  OutDataTypeStr=uint8  SaturateOnIntegerOverflow=off  RndMeth=Floor
  Data Type Conversion4 : DataTypeConversion  OutDataTypeStr=uint32  SaturateOnIntegerOverflow=off  RndMeth=Floor
  Terminator : Terminator
  CRC : Outport  OutDataTypeStr=uint8
  payload : Outport  Port=2  OutDataTypeStr=uint32
  error : Outport  Port=3  OutDataTypeStr=boolean
  wires:
  DATA/1 -> Terminator/1, Bit Slice1/1, Bit Slice4/1, Bit Slice3/1
  Bit Slice3/1 -> Data Type Conversion3/1
  Bit Slice4/1 -> Data Type Conversion4/1
  Data Type Conversion3/1 -> CRC/1
  Data Type Conversion4/1 -> payload/1
  Bit Slice1/1 -> Data Type Conversion1/1
  Data Type Conversion1/1 -> error/1

== system UZ_EnDat_be4_optimizing_agaib/UZ_ENDAT/RESPONSESLICER3X/25BITSLICER/responseslicer ==
  DATA : Inport  OutDataTypeStr=uint64
  Bit Slice1 : hdlsllib/Logic and Bit Operations/Bit Slice  lidx=2  ridx=2
  Bit Slice3 : hdlsllib/Logic and Bit Operations/Bit Slice  lidx=31  ridx=27
  Bit Slice4 : hdlsllib/Logic and Bit Operations/Bit Slice  lidx=26  ridx=2
  Data Type Conversion1 : DataTypeConversion  OutDataTypeStr=boolean  SaturateOnIntegerOverflow=off  RndMeth=Floor
  Data Type Conversion3 : DataTypeConversion  OutDataTypeStr=uint8  SaturateOnIntegerOverflow=off  RndMeth=Floor
  Data Type Conversion4 : DataTypeConversion  OutDataTypeStr=uint32  SaturateOnIntegerOverflow=off  RndMeth=Floor
  Terminator : Terminator
  CRC : Outport  OutDataTypeStr=uint8
  payload : Outport  Port=2  OutDataTypeStr=uint32
  error : Outport  Port=3  OutDataTypeStr=boolean
  wires:
  DATA/1 -> Terminator/1, Bit Slice1/1, Bit Slice4/1, Bit Slice3/1
  Bit Slice3/1 -> Data Type Conversion3/1
  Bit Slice4/1 -> Data Type Conversion4/1
  Data Type Conversion3/1 -> CRC/1
  Data Type Conversion4/1 -> payload/1
  Bit Slice1/1 -> Data Type Conversion1/1
  Data Type Conversion1/1 -> error/1

== system UZ_EnDat_be4_optimizing_agaib/UZ_ENDAT/RESPONSESLICER3X/25BITSLICER/responseslicer1 ==
  DATA : Inport  OutDataTypeStr=uint64
  Bit Slice1 : hdlsllib/Logic and Bit Operations/Bit Slice  lidx=2  ridx=2
  Bit Slice3 : hdlsllib/Logic and Bit Operations/Bit Slice  lidx=31  ridx=27
  Bit Slice4 : hdlsllib/Logic and Bit Operations/Bit Slice  lidx=26  ridx=2
  Data Type Conversion1 : DataTypeConversion  OutDataTypeStr=boolean  SaturateOnIntegerOverflow=off  RndMeth=Floor
  Data Type Conversion3 : DataTypeConversion  OutDataTypeStr=uint8  SaturateOnIntegerOverflow=off  RndMeth=Floor
  Data Type Conversion4 : DataTypeConversion  OutDataTypeStr=uint32  SaturateOnIntegerOverflow=off  RndMeth=Floor
  Terminator : Terminator
  CRC : Outport  OutDataTypeStr=uint8
  payload : Outport  Port=2  OutDataTypeStr=uint32
  error : Outport  Port=3  OutDataTypeStr=boolean
  wires:
  DATA/1 -> Terminator/1, Bit Slice1/1, Bit Slice4/1, Bit Slice3/1
  Bit Slice3/1 -> Data Type Conversion3/1
  Bit Slice4/1 -> Data Type Conversion4/1
  Data Type Conversion3/1 -> CRC/1
  Data Type Conversion4/1 -> payload/1
  Bit Slice1/1 -> Data Type Conversion1/1
  Data Type Conversion1/1 -> error/1

== system UZ_EnDat_be4_optimizing_agaib/UZ_ENDAT/RESPONSESLICER3X/25BITSLICER/responseslicer2 ==
  DATA : Inport  OutDataTypeStr=uint64
  Bit Slice1 : hdlsllib/Logic and Bit Operations/Bit Slice  lidx=2  ridx=2
  Bit Slice3 : hdlsllib/Logic and Bit Operations/Bit Slice  lidx=31  ridx=27
  Bit Slice4 : hdlsllib/Logic and Bit Operations/Bit Slice  lidx=26  ridx=2
  Data Type Conversion1 : DataTypeConversion  OutDataTypeStr=boolean  SaturateOnIntegerOverflow=off  RndMeth=Floor
  Data Type Conversion3 : DataTypeConversion  OutDataTypeStr=uint8  SaturateOnIntegerOverflow=off  RndMeth=Floor
  Data Type Conversion4 : DataTypeConversion  OutDataTypeStr=uint32  SaturateOnIntegerOverflow=off  RndMeth=Floor
  Terminator : Terminator
  CRC : Outport  OutDataTypeStr=uint8
  payload : Outport  Port=2  OutDataTypeStr=uint32
  error : Outport  Port=3  OutDataTypeStr=boolean
  wires:
  DATA/1 -> Terminator/1, Bit Slice1/1, Bit Slice4/1, Bit Slice3/1
  Bit Slice3/1 -> Data Type Conversion3/1
  Bit Slice4/1 -> Data Type Conversion4/1
  Data Type Conversion3/1 -> CRC/1
  Data Type Conversion4/1 -> payload/1
  Bit Slice1/1 -> Data Type Conversion1/1
  Data Type Conversion1/1 -> error/1

== system UZ_EnDat_be4_optimizing_agaib/UZ_ENDAT/RESPONSESLICER3X/27BITSLICER/responseslicer ==
  DATA : Inport  OutDataTypeStr=uint64
  Bit Slice1 : hdlsllib/Logic and Bit Operations/Bit Slice  lidx=2  ridx=2
  Bit Slice3 : hdlsllib/Logic and Bit Operations/Bit Slice  lidx=33  ridx=29
  Bit Slice4 : hdlsllib/Logic and Bit Operations/Bit Slice  lidx=28  ridx=2
  Data Type Conversion1 : DataTypeConversion  OutDataTypeStr=boolean  SaturateOnIntegerOverflow=off  RndMeth=Floor
  Data Type Conversion3 : DataTypeConversion  OutDataTypeStr=uint8  SaturateOnIntegerOverflow=off  RndMeth=Floor
  Data Type Conversion4 : DataTypeConversion  OutDataTypeStr=uint32  SaturateOnIntegerOverflow=off  RndMeth=Floor
  Terminator : Terminator
  CRC : Outport  OutDataTypeStr=uint8
  payload : Outport  Port=2  OutDataTypeStr=uint32
  error : Outport  Port=3  OutDataTypeStr=boolean
  wires:
  DATA/1 -> Terminator/1, Bit Slice1/1, Bit Slice4/1, Bit Slice3/1
  Bit Slice3/1 -> Data Type Conversion3/1
  Bit Slice4/1 -> Data Type Conversion4/1
  Data Type Conversion3/1 -> CRC/1
  Data Type Conversion4/1 -> payload/1
  Bit Slice1/1 -> Data Type Conversion1/1
  Data Type Conversion1/1 -> error/1

== system UZ_EnDat_be4_optimizing_agaib/UZ_ENDAT/RESPONSESLICER3X/27BITSLICER/responseslicer1 ==
  DATA : Inport  OutDataTypeStr=uint64
  Bit Slice1 : hdlsllib/Logic and Bit Operations/Bit Slice  lidx=2  ridx=2
  Bit Slice3 : hdlsllib/Logic and Bit Operations/Bit Slice  lidx=33  ridx=29
  Bit Slice4 : hdlsllib/Logic and Bit Operations/Bit Slice  lidx=28  ridx=2
  Data Type Conversion1 : DataTypeConversion  OutDataTypeStr=boolean  SaturateOnIntegerOverflow=off  RndMeth=Floor
  Data Type Conversion3 : DataTypeConversion  OutDataTypeStr=uint8  SaturateOnIntegerOverflow=off  RndMeth=Floor
  Data Type Conversion4 : DataTypeConversion  OutDataTypeStr=uint32  SaturateOnIntegerOverflow=off  RndMeth=Floor
  Terminator : Terminator
  CRC : Outport  OutDataTypeStr=uint8
  payload : Outport  Port=2  OutDataTypeStr=uint32
  error : Outport  Port=3  OutDataTypeStr=boolean
  wires:
  DATA/1 -> Terminator/1, Bit Slice1/1, Bit Slice4/1, Bit Slice3/1
  Bit Slice3/1 -> Data Type Conversion3/1
  Bit Slice4/1 -> Data Type Conversion4/1
  Data Type Conversion3/1 -> CRC/1
  Data Type Conversion4/1 -> payload/1
  Bit Slice1/1 -> Data Type Conversion1/1
  Data Type Conversion1/1 -> error/1

== system UZ_EnDat_be4_optimizing_agaib/UZ_ENDAT/RESPONSESLICER3X/27BITSLICER/responseslicer2 ==
  DATA : Inport  OutDataTypeStr=uint64
  Bit Slice1 : hdlsllib/Logic and Bit Operations/Bit Slice  lidx=2  ridx=2
  Bit Slice3 : hdlsllib/Logic and Bit Operations/Bit Slice  lidx=33  ridx=29
  Bit Slice4 : hdlsllib/Logic and Bit Operations/Bit Slice  lidx=28  ridx=2
  Data Type Conversion1 : DataTypeConversion  OutDataTypeStr=boolean  SaturateOnIntegerOverflow=off  RndMeth=Floor
  Data Type Conversion3 : DataTypeConversion  OutDataTypeStr=uint8  SaturateOnIntegerOverflow=off  RndMeth=Floor
  Data Type Conversion4 : DataTypeConversion  OutDataTypeStr=uint32  SaturateOnIntegerOverflow=off  RndMeth=Floor
  Terminator : Terminator
  CRC : Outport  OutDataTypeStr=uint8
  payload : Outport  Port=2  OutDataTypeStr=uint32
  error : Outport  Port=3  OutDataTypeStr=boolean
  wires:
  DATA/1 -> Terminator/1, Bit Slice1/1, Bit Slice4/1, Bit Slice3/1
  Bit Slice3/1 -> Data Type Conversion3/1
  Bit Slice4/1 -> Data Type Conversion4/1
  Data Type Conversion3/1 -> CRC/1
  Data Type Conversion4/1 -> payload/1
  Bit Slice1/1 -> Data Type Conversion1/1
  Data Type Conversion1/1 -> error/1

== system UZ_EnDat_be4_optimizing_agaib/UZ_ENDAT/Subsystem/stalebootupfunction/CLKCNTERBOOTUP ==
  CLK : Inport
  CLK2CNT : Inport  Port=2
  ResetCNT : Inport  Port=3  OutDataTypeStr=boolean
  Delay1 : Delay  DelayLength=1
  Positional_Counter : Subsystem  TreatAsAtomicUnit=on
      settings: LibrarySourceBlock=|
      | hdlsllib/Ports &
      | Subsystems/Triggered
      | Subsystem
  SetZero32modified : Subsystem
  CNT : Outport
  wires:
  CLK2CNT/1 -> Positional_Counter/Trigger
  Delay1/1 -> Positional_Counter/1(valueout), CNT/1
  SetZero32modified/1(valueout) -> Delay1/1
  CLK/1 -> SetZero32modified/Trigger
  Positional_Counter/1(divider) -> SetZero32modified/1(valin)
  ResetCNT/1 -> SetZero32modified/2(setzero)

== system UZ_EnDat_be4_optimizing_agaib/UZ_ENDAT/Subsystem/stalebootupfunction/ManualDeserializere ==
  CLK : Inport
  SLOWCLCK : Inport  Port=2
  DATA : Inport  Port=3
  reset : Inport  Port=4
  14 : Inport  Port=5
  Constant3 : Constant  Value=0  OutDataTypeStr=boolean  SampleTime=-1
  Data Type Conversion : DataTypeConversion  OutMin=0  OutMax=1  OutDataTypeStr=fixdt(0,1)  SaturateOnIntegerOverflow=off  RndMeth=Floor
  Delay : Delay  DelayLength=1
  Delay1 : Delay  DelayLength=1
  Logical Operator : Logic  Operator=NOT  AllPortsSameDT=off  OutDataTypeStr=boolean
  Multiport Switch : MultiPortSwitch  Inputs=16  DataPortForDefault=Additional data port  DiagnosticForDefault=None  SaturateOnIntegerOverflow=off  InputSameDT=off
  Switch : Switch  Criteria=u2 ~= 0  SaturateOnIntegerOverflow=off  InputSameDT=off
  WORDTOBOOL : Subsystem  TreatAsAtomicUnit=on
  ramwatcher : Subsystem  TreatAsAtomicUnit=on
      settings: LibrarySourceBlock=|
      | hdlsllib/Ports &
      | Subsystems/Triggered
      | Subsystem
  valin : Outport
  wires:
  SLOWCLCK/1 -> Switch/1, Delay/1
  DATA/1 -> WORDTOBOOL/1(DATAIN)
  Multiport Switch/1 -> valin/1
  CLK/1 -> WORDTOBOOL/Trigger
  Delay1/1 -> ramwatcher/1(In1)
  Constant3/1 -> Multiport Switch/18
  reset/1 -> Logical Operator/1
  Logical Operator/1 -> Data Type Conversion/1
  Data Type Conversion/1 -> ramwatcher/2(In2)
  WORDTOBOOL/1(DATAOUT0) -> Multiport Switch/17
  WORDTOBOOL/2(DATAOUT1) -> Multiport Switch/16
  WORDTOBOOL/3(DATAOUT2) -> Multiport Switch/15
  WORDTOBOOL/4(DATAOUT3) -> Multiport Switch/14
  WORDTOBOOL/5(DATAOUT4) -> Multiport Switch/13
  WORDTOBOOL/6(DATAOUT5) -> Multiport Switch/12
  WORDTOBOOL/9(DATAOUT8) -> Multiport Switch/9
  WORDTOBOOL/10(DATAOUT9) -> Multiport Switch/8
  WORDTOBOOL/11(DATAOUT10) -> Multiport Switch/7
  WORDTOBOOL/12(DATAOUT11) -> Multiport Switch/6
  WORDTOBOOL/13(DATAOUT12) -> Multiport Switch/5
  WORDTOBOOL/14(DATAOUT13) -> Multiport Switch/4
  WORDTOBOOL/15(DATAOUT14) -> Multiport Switch/3
  WORDTOBOOL/16(DATAOUT15) -> Multiport Switch/2
  WORDTOBOOL/7(DATAOUT6) -> Multiport Switch/11
  WORDTOBOOL/8(DATAOUT7) -> Multiport Switch/10
  14/1 -> Switch/2
  ramwatcher/1(SEL) -> Multiport Switch/1, Delay1/1
  Switch/1 -> ramwatcher/Trigger
  Delay/1 -> Switch/3
